simulink model "p3"  (R2020b)
settings: Solver=VariableStepAuto  StartTime=0.0  StopTime=10.0  RelTol=1e-3
model workspace (MAT data in the model file):
  A = 0.5792
  B = -0.5792
  C = 0.158
settings Model: Creator=DELL  LastModifiedBy=DELL

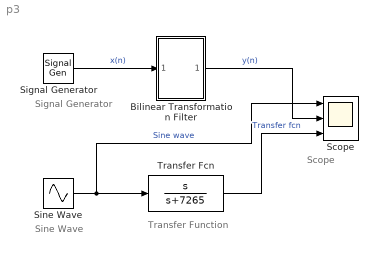
== system p3 ==
  note: Transfer Function
  note: Sine Wave
  note: Signal
      | Generator
  note: Scope
  Bilinear Transformation Filter : Subsystem
  Scope : Scope  NumInputPorts=3
  Signal Generator : SignalGenerator  Units=rad/sec
  Sine Wave : Sin  Frequency=3455.75  SampleTime=0
  Transfer Fcn : TransferFcn  Numerator=[1 0]  Denominator=[1 7265]
  wires:
  Transfer Fcn/1 -> Scope/3  "Transfer fcn"
  Bilinear Transformation Filter/1(y(n)) -> Scope/2  "y(n)"
  Sine Wave/1 -> Scope/1, Transfer Fcn/1  "Sine wave"
  Signal Generator/1 -> Bilinear Transformation Filter/1(x(n))  "x(n)"

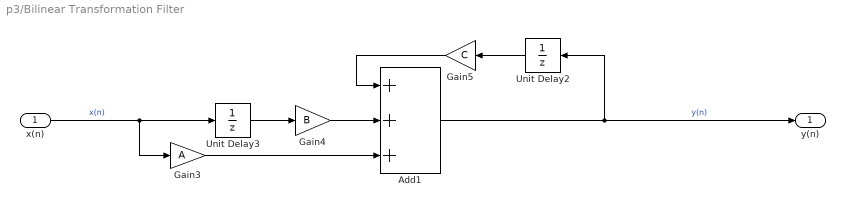
== system p3/Bilinear Transformation Filter ==
  x(n) : Inport
  Add1 : Sum  Inputs=+++
  Gain3 : Gain  Gain=A
  Gain4 : Gain  Gain=B
  Gain5 : Gain  Gain=C
  Unit Delay2 : UnitDelay  SampleTime=-1  HasFrameUpgradeWarning=on
  Unit Delay3 : UnitDelay  SampleTime=-1  HasFrameUpgradeWarning=on
  y(n) : Outport
  wires:
  Unit Delay3/1 -> Gain4/1
  Gain5/1 -> Add1/1
  Add1/1 -> y(n)/1, Unit Delay2/1  "y(n)"
  Gain3/1 -> Add1/3
  Gain4/1 -> Add1/2
  Unit Delay2/1 -> Gain5/1
  x(n)/1 -> Gain3/1, Unit Delay3/1  "x(n)"
